simulink subsystem "Aerodinamicaa"  (R2021b)
settings: Solver=VariableStepAuto  StartTime=0.0  StopTime=10.0  RelTol=1e-3
values from neighbouring files (symbols this model uses):
  b_ala = 3    [aerodinamica.m]    (also in codigos.m; help.mat)
  b_est = 1    [aerodinamica.m]    (also in codigos.m; help.mat)
  c = 0.2    [aerodinamica.m]    (also in codigos.m; help.mat)
  Cd0 = 0.045    [aerodinamica.m]    (also in codigos.m; help.mat)
  CL0 = 0.25    [aerodinamica.m]    (also in codigos.m; help.mat)
  Cl_deltaa = 0.17    [aerodinamica.m]    (also in codigos.m; help.mat)
  Cl_p = 0.51    [aerodinamica.m]    (also in codigos.m; help.mat)
  CLalpha = 5.5    [codigos.m]    (also in help.mat)
  Cm_deltae = 1    [aerodinamica.m]    (also in codigos.m; help.mat)
  Cm_fq = 0.1    [aerodinamica.m]    (also in codigos.m; help.mat)
  Cm_w = 0.0005    [aerodinamica.m]    (also in codigos.m; help.mat)
  Cn_deltar = 0.07    [aerodinamica.m]    (also in codigos.m; help.mat)
  Cn_fr = 0.1    [aerodinamica.m]    (also in codigos.m; help.mat)
  Cn_v = 0.002    [aerodinamica.m]    (also in codigos.m; help.mat)
  e = 0.75    [aerodinamica.m]    (also in codigos.m; help.mat)
  g = 9.80665    [aerodinamica.m]    (also in codigos.m; eom.m; help.mat)
  h = 0.7    [aerodinamica.m]    (also in codigos.m; help.mat)
  L_ala = 0.25    [aerodinamica.m]    (also in codigos.m; help.mat)
  L_est = 0.1    [aerodinamica.m]    (also in codigos.m; help.mat)
  Long = 2    [aerodinamica.m]    (also in codigos.m; help.mat)
  m = 15    [aerodinamica.m]    (also in codigos.m; eom.m; help.mat)
settings Model: DefaultTestHarness=Misil_Simulink_Harness1  Creator=verti  LastModifiedBy=verti

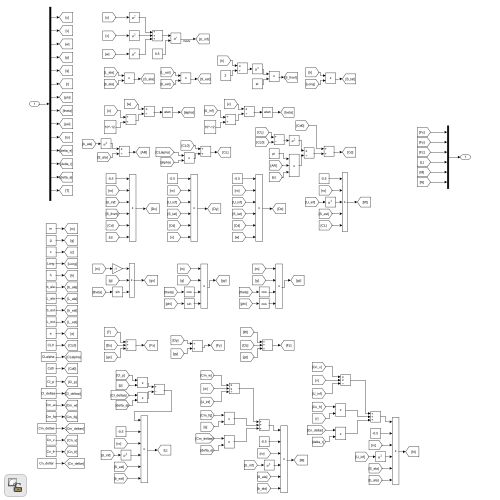
[thumbnail: Simulink's stored preview of the top-level diagram]
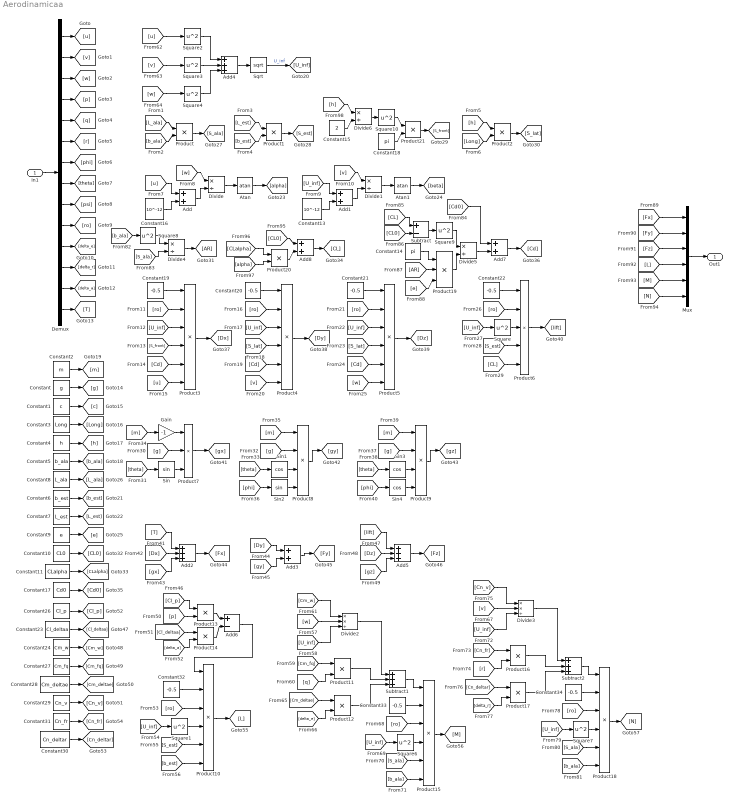
== system Aerodinamicaa ==
  In1 : Inport
  Add{,1,3,7..8} (5 alike) : Sum
  Add2 : Sum  Inputs=+++
  Add4 : Sum  Inputs=+++
  Add5 : Sum  Inputs=+++
  Add6 : Sum  Inputs=+-
  Atan : Trigonometry  Operator=atan
  Atan1 : Trigonometry  Operator=atan
  Constant : Constant  Value=g
  Constant1 : Constant  Value=c
  Constant10 : Constant  Value=CL0
  Constant11 : Constant  Value=CLalpha
  Constant13 : Constant  Value=10^-12
  Constant14 : Constant  Value=pi
  Constant15 : Constant  Value=2
  Constant16 : Constant  Value=10^-12
  Constant17 : Constant  Value=Cd0
  Constant18 : Constant  Value=pi
  Constant{19..22,32..34} (7 alike) : Constant  Value=-0.5
  Constant2 : Constant  Value=m
  Constant23 : Constant  Value=Cl_deltaa
  Constant24 : Constant  Value=Cm_w
  Constant26 : Constant  Value=Cl_p
  Constant27 : Constant  Value=Cm_fq
  Constant28 : Constant  Value=Cm_deltae
  Constant29 : Constant  Value=Cn_v
  Constant3 : Constant  Value=Long
  Constant30 : Constant  Value=Cn_deltar
  Constant31 : Constant  Value=Cn_fr
  Constant4 : Constant  Value=h
  Constant5 : Constant  Value=b_ala
  Constant6 : Constant  Value=b_est
  Constant7 : Constant  Value=L_est
  Constant8 : Constant  Value=L_ala
  Constant9 : Constant  Value=e
  Demux : Demux  Outputs=14
  Divide{,1,4..6} (5 alike) : Product  Inputs=*/
  Divide2 : Product  Inputs=**/
  Divide3 : Product  Inputs=**/
  Gain : Gain  Gain=-1
  Mux : Mux  Inputs=6
  Product{,1..2,11..14,16..17,20..21} (11 alike) : Product
  Product{3..5,10,15,18} (6 alike) : Product  Inputs=6
  Product19 : Product  Inputs=3
  Product6 : Product  Inputs=5
  Product7 : Product  Inputs=3
  Product8 : Product  Inputs=4
  Product9 : Product  Inputs=4
  Sin : Trigonometry
  Sin1 : Trigonometry  Operator=cos
  Sin2 : Trigonometry
  Sin3 : Trigonometry  Operator=cos
  Sin4 : Trigonometry  Operator=cos
  Sqrt : Sqrt  SaturateOnIntegerOverflow=on
  Square{,1..4,6..10} (10 alike) : Math  Operator=square  SaturateOnIntegerOverflow=on
  Subtract : Sum  Inputs=+-
  Subtract1 : Sum  Inputs=+++
  Subtract2 : Sum  Inputs=+++
  Out1 : Outport
  wires:
  In1/1 -> Demux/1
  Mux/1 -> Out1/1
  Demux/1 -> [u]
  Demux/2 -> [v]
  Demux/6 -> [r]
  Demux/5 -> [q]
  Demux/4 -> [p]
  Demux/3 -> [w]
  Demux/7 -> [phi]
  Demux/14 -> [T]
  Demux/13 -> [delta_a]
  Demux/12 -> [delta_r]
  Demux/11 -> [delta_e]
  Demux/10 -> [ro]
  Demux/9 -> [psi]
  Demux/8 -> [theta]
  Constant3/1 -> [Long]
  Constant2/1 -> [m]
  Constant/1 -> [g]
  Constant4/1 -> [h]
  Constant5/1 -> [b_ala]
  Constant1/1 -> [c]
  Add4/1 -> Sqrt/1
  Sqrt/1 -> [U_inf]  "U_inf"
  Square3/1 -> Add4/2
  [w] -> Square4/1
  [v] -> Square3/1
  Square4/1 -> Add4/3
  Square2/1 -> Add4/1
  [u] -> Square2/1
  Constant7/1 -> [L_est]
  Constant11/1 -> [CLalpha]
  Constant10/1 -> [CL0]
  Constant6/1 -> [b_est]
  Constant9/1 -> [e]
  [L_ala] -> Product/1
  [b_ala] -> Product/2
  Product/1 -> [S_ala]
  Product1/1 -> [S_est]
  [b_est] -> Product1/2
  [L_est] -> Product1/1
  [h] -> Product2/1
  Product2/1 -> [S_lat]
  [Long] -> Product2/2
  [u] -> Add/1
  Divide/1 -> Atan/1
  Add/1 -> Divide/2
  Atan/1 -> [alpha]
  [w] -> Divide/1
  Constant16/1 -> Add/2
  Constant13/1 -> Add1/2
  [v] -> Divide1/1
  Atan1/1 -> [beta]
  Add1/1 -> Divide1/2
  Divide1/1 -> Atan1/1
  [U_inf] -> Add1/1
  Divide4/1 -> [AR]
  Constant17/1 -> [Cd0]
  [U_inf] -> Product3/3
  [ro] -> Product3/2
  [Cd] -> Product3/5
  Constant19/1 -> Product3/1
  Product3/1 -> [Dx]
  [u] -> Product3/6
  [S_front] -> Product3/4
  [S_lat] -> Product4/4
  [v] -> Product4/6
  Product4/1 -> [Dy]
  Constant20/1 -> Product4/1
  [Cd] -> Product4/5
  [ro] -> Product4/2
  [U_inf] -> Product4/3
  [U_inf] -> Product5/3
  [ro] -> Product5/2
  [Cd] -> Product5/5
  Constant21/1 -> Product5/1
  Product5/1 -> [Dz]
  [w] -> Product5/6
  [S_lat] -> Product5/4
  [S_est] -> Product6/4
  Product6/1 -> [lift]
  Constant22/1 -> Product6/1
  [CL] -> Product6/5
  [ro] -> Product6/2
  [U_inf] -> Square/1
  Square/1 -> Product6/3
  Gain/1 -> Product7/1
  [g] -> Product7/2
  [theta] -> Sin/1
  Sin/1 -> Product7/3
  Product7/1 -> [gx]
  Product8/1 -> [gy]
  Sin1/1 -> Product8/3
  [theta] -> Sin1/1
  [g] -> Product8/2
  [m] -> Product8/1
  [m] -> Gain/1
  [phi] -> Sin2/1
  Sin2/1 -> Product8/4
  Sin4/1 -> Product9/4
  [phi] -> Sin4/1
  [m] -> Product9/1
  [g] -> Product9/2
  [theta] -> Sin3/1
  Sin3/1 -> Product9/3
  Product9/1 -> [gz]
  [T] -> Add2/1
  [Dx] -> Add2/2
  [gx] -> Add2/3
  Add2/1 -> [Fx]
  [gy] -> Add3/2
  Add3/1 -> [Fy]
  [Dy] -> Add3/1
  [lift] -> Add5/1
  Add5/1 -> [Fz]
  [gz] -> Add5/3
  [Dz] -> Add5/2
  Constant30/1 -> [Cn_deltar]
  Constant24/1 -> [Cm_w]
  Constant29/1 -> [Cn_v]
  Constant28/1 -> [Cm_deltae]
  Constant23/1 -> [Cl_deltaa]
  Constant26/1 -> [Cl_p]
  Constant27/1 -> [Cm_fq]
  Constant31/1 -> [Cn_fr]
  [Cl_p] -> Product13/1
  Product14/1 -> Add6/2
  [Cl_deltaa] -> Product14/1
  [p] -> Product13/2
  [delta_a] -> Product14/2
  [ro] -> Product10/3
  Square1/1 -> Product10/4
  [b_est] -> Product10/6
  Constant32/1 -> Product10/2
  Add6/1 -> Product10/1
  [U_inf] -> Square1/1
  Product10/1 -> [L]
  Product13/1 -> Add6/1
  [S_est] -> Product10/5
  Product15/1 -> [M]
  [Cm_fq] -> Product11/1
  [Cm_w] -> Divide2/1
  [S_ala] -> Product15/5
  [U_inf] -> Square6/1
  Divide2/1 -> Subtract1/1
  [w] -> Divide2/2
  [b_ala] -> Product15/6
  [ro] -> Product15/3
  Subtract1/1 -> Product15/1
  [U_inf] -> Divide2/3
  Constant33/1 -> Product15/2
  Product11/1 -> Subtract1/2
  [q] -> Product11/2
  Square6/1 -> Product15/4
  [delta_e] -> Product12/2
  [Cm_deltae] -> Product12/1
  Product12/1 -> Subtract1/3
  Product17/1 -> Subtract2/3
  [Cn_deltar] -> Product17/1
  [delta_r] -> Product17/2
  Square7/1 -> Product18/4
  [r] -> Product16/2
  Product16/1 -> Subtract2/2
  Constant34/1 -> Product18/2
  [U_inf] -> Divide3/3
  Subtract2/1 -> Product18/1
  [ro] -> Product18/3
  [b_ala] -> Product18/6
  [v] -> Divide3/2
  Divide3/1 -> Subtract2/1
  [U_inf] -> Square7/1
  [S_ala] -> Product18/5
  [Cn_v] -> Divide3/1
  [Cn_fr] -> Product16/1
  Product18/1 -> [N]
  [b_ala] -> Square8/1
  [S_ala] -> Divide4/2
  Square8/1 -> Divide4/1
  Add7/1 -> [Cd]
  [Cd0] -> Add7/1
  [CL0] -> Subtract/2
  [CL] -> Subtract/1
  Subtract/1 -> Square9/1
  Square9/1 -> Divide5/1
  Product19/1 -> Divide5/2
  Constant14/1 -> Product19/1
  [AR] -> Product19/2
  [e] -> Product19/3
  Divide5/1 -> Add7/2
  [Fx] -> Mux/1
  [Fy] -> Mux/2
  [Fz] -> Mux/3
  [L] -> Mux/4
  [M] -> Mux/5
  [N] -> Mux/6
  Add8/1 -> [CL]
  Product20/1 -> Add8/2
  [CL0] -> Add8/1
  [alpha] -> Product20/2
  [CLalpha] -> Product20/1
  [h] -> Divide6/1
  Constant15/1 -> Divide6/2
  Product21/1 -> [S_front]
  Divide6/1 -> Square10/1
  Constant18/1 -> Product21/2
  Square10/1 -> Product21/1
  Constant8/1 -> [L_ala]
